simulink model "example_Hydraulic_ValveThermostatic"  (R2016b)
settings: Solver=ode45  StartTime=0.0  StopTime=600  RelTol=1e-3  EnableMultiTasking=on
undefined symbols (not defined in the file): path_carnot
libraries: carnot x6
settings Model: Creator=drhf  LastModifiedBy=drhf
settings DataIOCC: LimitDataPoints=on  SaveFormat=Array  SignalLoggingSaveFormat=ModelDataLogs
settings OptimizationCC: ExpressionDepthLimit=2147483647  LifeSpan=inf
settings DebuggingCC: UnderspecifiedInitializationDetection=Classic  MergeDetectMultiDrivingBlocksExec=none  SolverPrmCheckMsg=warning  FcnCallInpInsideContextMsg=warning  StateNameClashWarn=warning  SFUnexpectedBacktrackingDiag=warning  SFNoUnconditionalDefaultTransitionDiag=warning  SFExecutionAtInitializationDiag=none
settings HardwareCC: ProdBitPerPointer=32  ProdBitPerSizeT=32  ProdBitPerPtrDiffT=32  ProdLargestAtomicFloat=None  ProdIntDivRoundTo=Undefined  ProdEndianess=Unspecified  ProdWordSize=32  ProdHWDeviceType=32-bit Generic
settings ModelReferenceCC: PropagateSignalLabelsOutOfModel=off
settings GRTTargetCC: TargetLangStandard=C89/C90 (ANSI)  GeneratePreprocessorConditionals=Disable all  CombineOutputUpdateFcns=off  GRTInterface=on
settings ConfigComp: CovMetricSettings=dw  CovHtmlReporting=on  CovSaveCumulativeToWorkspaceVar=on  CovSaveSingleToWorkspaceVar=on  CovExternalEMLEnable=off

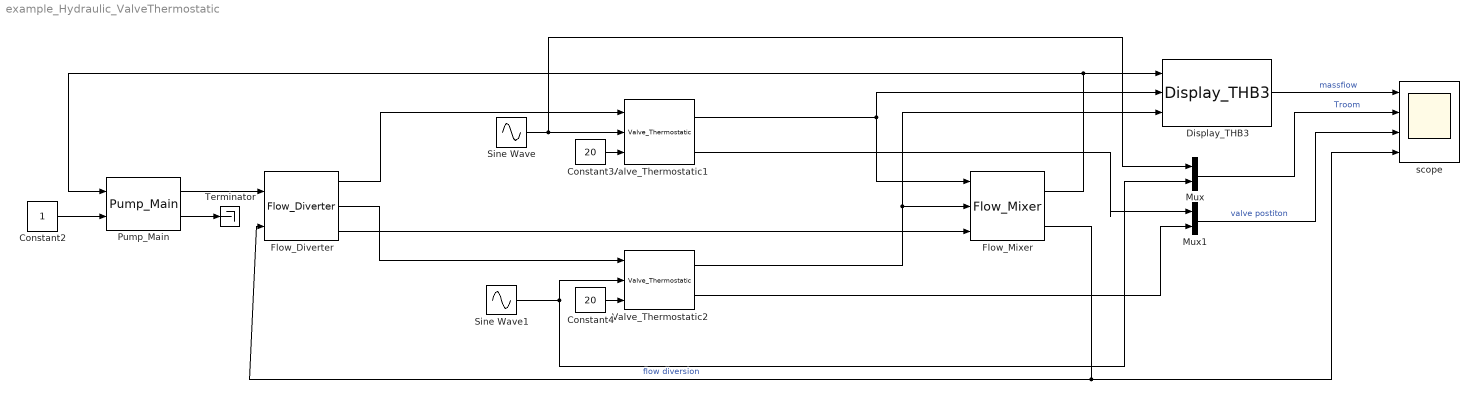
== system example_Hydraulic_ValveThermostatic ==
  Constant2 : Constant
  Constant3 : Constant  Value=20
  Constant4 : Constant  Value=20
  Display_THB3 : carnot/Outputs/Display_THB3  t=off  m=on  p=off  id=off  mix=off  d=off
  Flow_Diverter : carnot/Hydraulics/Flow_Diverter
  Flow_Mixer : carnot/Hydraulics/Flow_Mixer  t=1
  Mux : Mux  Inputs=2
  Mux1 : Mux  Inputs=2
  Pump_Main : carnot/Hydraulics/Pump_Main  Tini=20  p0=3e5  IDpreset=pressure drop  fluid=Water  mix=0  mix2=0  mix3=0  t1=1  PathName=fullfile(path_carnot('libsl'), 'Hydraulics', 'Pump_Main', 'parameter_set')  FileName='Pump6m.mat'  userPath=off  userParam=off  a0=60000  a1=-43200  a2=0  dia=0.025  UA=1  mcp=4182  e0=50  e1=28.8  e2=-10.368
  Sine Wave : Sin  Amplitude=4  Bias=20  Frequency=1/60  SampleTime=0
  Sine Wave1 : Sin  Amplitude=4  Bias=20  Frequency=1/60  Phase=pi  SampleTime=0
  Terminator : Terminator
  Valve_Thermostatic1 : carnot/Hydraulics/Valve_Thermostatic  p=4  op=0.5  bl=0.1  ts=1  dt_V=1  ART=linear  kvs=2  psi_0=0.04
  Valve_Thermostatic2 : carnot/Hydraulics/Valve_Thermostatic  p=4  op=0.5  bl=0.1  ts=1  dt_V=1  ART=linear  kvs=2  psi_0=0.04
  scope : Scope  NumInputPorts=4
  wires:
  Constant2/1 -> Pump_Main/2
  Pump_Main/2 -> Terminator/1
  Sine Wave/1 -> Mux/1, Valve_Thermostatic1/2
  Pump_Main/1 -> Flow_Diverter/1
  Flow_Diverter/1 -> Valve_Thermostatic1/1
  Sine Wave1/1 -> Mux/2, Valve_Thermostatic2/2
  Flow_Diverter/2 -> Valve_Thermostatic2/1
  Flow_Diverter/3 -> Flow_Mixer/3
  Flow_Mixer/2 -> scope/4, Flow_Diverter/2  "flow diversion"
  Flow_Mixer/1 -> Pump_Main/1, Display_THB3/1
  Display_THB3/1 -> scope/1  "massfiow"
  Mux1/1 -> scope/3  "valve postiton"
  Valve_Thermostatic2/1 -> Flow_Mixer/2, Display_THB3/3
  Valve_Thermostatic1/1 -> Flow_Mixer/1, Display_THB3/2
  Valve_Thermostatic1/2 -> Mux1/1
  Valve_Thermostatic2/2 -> Mux1/2
  Constant3/1 -> Valve_Thermostatic1/3
  Constant4/1 -> Valve_Thermostatic2/3
  Mux/1 -> scope/2  "Troom"
